simulink model "Control_UAV_Phat"  (R2016a)
settings: Solver=VariableStepAuto  StartTime=0.0  StopTime=30  RelTol=1e-3
PreLoadFcn:
  | parameters
InitFcn:
  | parameters
values from neighbouring files (symbols this model uses):
  attitudeInit = [0;0;0]    [parameters.m]
  b = 5.9347e-06    [parameters.m]
  d = 1.2181e-07    [parameters.m]
  g = 9.81    [parameters.m]
  I = diag([Ix,Iy,Iz])    [parameters.m]
  k1_pitch = kxip*wp_n*Iy/(Kth*L)    [parameters.m]
  k1_roll = kxir*wr_n*Ix/(Kth*L)    [parameters.m]
  k1_yaw = kxiy*wy_n*Iz/(2*Kd)    [parameters.m]
  k2_pitch = (wp_n^2)*Iy/(2*k1_pitch*Kth*L)    [parameters.m]
  k2_roll = (wr_n^2)*Ix/(2*k1_roll*Kth*L)    [parameters.m]
  k2_yaw = (wy_n^2)*Iz/(4*k1_yaw*Kd)    [parameters.m]
  kd_x = 4*g/(kxi_positionx*wposition_nx)    (= 29.0666666667)    [parameters.m]
  kd_y = 4*g/(kxi_positiony*wposition_ny)    (= 78.48)    [parameters.m]
  ki_h = 0.04    [parameters.m]
  kp_h = 2*wh_n*kxih*m/(4*Kth)    [parameters.m]
  kp_x = 2*g/wposition_nx^2    (= 8.72)    [parameters.m]
  kp_y = 2*g/wposition_ny^2    (= 19.62)    [parameters.m]
  Ks = 735    [parameters.m]
  L = 0.17    [parameters.m]
  m = 0.616    [parameters.m]
  omegaInit = [0;0;0]    [parameters.m]
  posInit = [0;0;0]    [parameters.m]
  tau = 1/200    (= 0.005)    [parameters.m]
  u0 = 0.49    [parameters.m]
  velInit = [0;0;0]    [parameters.m]
settings Model: Creator=Hiii  LastModifiedBy=Hii
settings GRTTargetCC: GeneratePreprocessorConditionals=Use local settings

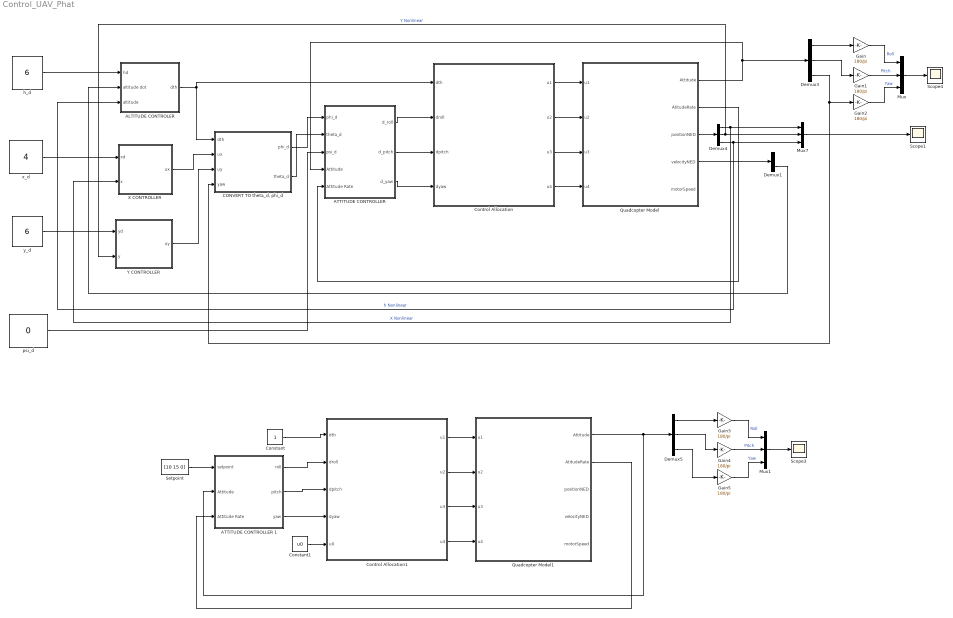
== system Control_UAV_Phat ==
  "ALTITUDE CONTROLER " : Subsystem
  "ATTITUDE CONTROLLER " : Subsystem
  ATTITUDE CONTROLLER 1 : Subsystem
  "CONVERT TO theta_d, phi_d " : MATLAB Function  TreatAsAtomicUnit=on
  Constant : Constant
  Constant1 : Constant  Value=u0
  Control Allocation : Subsystem
  Control Allocation1 : Subsystem
  Demux{1,3..5} (4 alike) : Demux  Outputs=3
  Gain{,1..5} (6 alike) : Gain  Gain=180/pi
  Mux : Mux  Inputs=3
  Mux1 : Mux  Inputs=3
  Mux7 : Mux  Inputs=3
  Quadcopter Model : Subsystem
  Quadcopter Model1 : Subsystem
  Scope1 : Scope
  Scope3 : Scope
  Scope4 : Scope
  "Setpoint " : Constant  Value=[10 15 0]
  "X CONTROLLER " : Subsystem
  "Y CONTROLLER " : Subsystem
  "h_d " : Constant  Value=6
  psi_d : Constant  Value=0
  "x_d " : Constant  Value=4
  "y_d " : Constant  Value=6
  wires:
  Demux3/3 -> Gain2/1, "CONVERT TO theta_d, phi_d "/4(yaw)
  Demux4/3 -> "ALTITUDE CONTROLER "/3("altitude "), Mux7/3  "h Nonlinear"
  Demux4/2 -> "Y CONTROLLER "/2(y), Mux7/2  "Y Nonlinear"
  Demux4/1 -> Mux7/1, "X CONTROLLER "/2(x)  "X Nonlinear"
  Quadcopter Model/3("positionNED ") -> Demux4/1
  Quadcopter Model/1(Attitude) -> "ATTITUDE CONTROLLER "/4("Attitude "), Demux3/1
  Quadcopter Model/4(velocityNED) -> Demux1/1
  "ALTITUDE CONTROLER "/1(dth) -> Control Allocation/1(dth), "CONVERT TO theta_d, phi_d "/1(dth)
  "X CONTROLLER "/1("ux ") -> "CONVERT TO theta_d, phi_d "/2(ux)
  "Y CONTROLLER "/1("uy ") -> "CONVERT TO theta_d, phi_d "/3(uy)
  "y_d "/1 -> "Y CONTROLLER "/1(yd)
  "x_d "/1 -> "X CONTROLLER "/1(xd)
  "h_d "/1 -> "ALTITUDE CONTROLER "/1(hd)
  Demux1/3 -> "ALTITUDE CONTROLER "/2("altitude dot ")
  Control Allocation/1("u1 ") -> Quadcopter Model/1("u1 ")
  Control Allocation/2("u2 ") -> Quadcopter Model/2("u2 ")
  Control Allocation/3("u3 ") -> Quadcopter Model/3("u3 ")
  Control Allocation/4("u4 ") -> Quadcopter Model/4("u4 ")
  "ATTITUDE CONTROLLER "/1("d_roll ") -> Control Allocation/2(droll)
  "ATTITUDE CONTROLLER "/2("d_pitch ") -> Control Allocation/3(dpitch)
  "ATTITUDE CONTROLLER "/3("d_yaw ") -> Control Allocation/4(dyaw)
  "CONVERT TO theta_d, phi_d "/1(phi_d) -> "ATTITUDE CONTROLLER "/1(phi_d)
  "CONVERT TO theta_d, phi_d "/2(theta_d) -> "ATTITUDE CONTROLLER "/2(theta_d)
  psi_d/1 -> "ATTITUDE CONTROLLER "/3("psi_d ")
  Quadcopter Model/2(AtitudeRate) -> "ATTITUDE CONTROLLER "/5("Attitude Rate ")
  Demux3/1 -> Gain/1
  Demux3/2 -> Gain1/1
  Mux/1 -> Scope4/1
  Gain/1 -> Mux/1  "Roll"
  Gain1/1 -> Mux/2  "Pitch"
  Gain2/1 -> Mux/3  "Yaw"
  Mux7/1 -> Scope1/1
  Demux5/3 -> Gain5/1
  Quadcopter Model1/1(Attitude) -> ATTITUDE CONTROLLER 1/2("Attitude "), Demux5/1
  Control Allocation1/1("u1 ") -> Quadcopter Model1/1("u1 ")
  Control Allocation1/2("u2 ") -> Quadcopter Model1/2("u2 ")
  Control Allocation1/3("u3 ") -> Quadcopter Model1/3("u3 ")
  Control Allocation1/4("u4 ") -> Quadcopter Model1/4("u4 ")
  ATTITUDE CONTROLLER 1/1("roll ") -> Control Allocation1/2(droll)
  ATTITUDE CONTROLLER 1/2("pitch ") -> Control Allocation1/3(dpitch)
  ATTITUDE CONTROLLER 1/3("yaw ") -> Control Allocation1/4(dyaw)
  Quadcopter Model1/2(AtitudeRate) -> ATTITUDE CONTROLLER 1/3("Attitude Rate ")
  Demux5/1 -> Gain3/1
  Demux5/2 -> Gain4/1
  Mux1/1 -> Scope3/1
  Gain3/1 -> Mux1/1  "Roll"
  Gain4/1 -> Mux1/2  "Pitch"
  Gain5/1 -> Mux1/3  "Yaw"
  Constant/1 -> Control Allocation1/1(dth)
  "Setpoint "/1 -> ATTITUDE CONTROLLER 1/1("setpoint ")
  Constant1/1 -> Control Allocation1/5("u0 ")

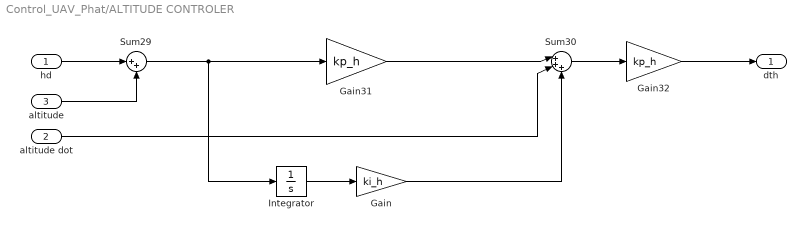
== system Control_UAV_Phat/ALTITUDE CONTROLER  ==
  hd : Inport  Description=hd
  "altitude dot " : Inport  Description=hd  Port=2
  "altitude " : Inport  Description=hd  Port=3
  Gain : Gain  Gain=ki_h
  Gain31 : Gain  Gain=kp_h
  Gain32 : Gain  Gain=kp_h
  Integrator : Integrator
  Sum29 : Sum  Inputs=|++
  Sum30 : Sum  Inputs=|+++
  dth : Outport
  wires:
  "altitude dot "/1 -> Sum30/2
  Sum30/1 -> Gain32/1
  Sum29/1 -> Integrator/1, Gain31/1
  hd/1 -> Sum29/1
  "altitude "/1 -> Sum29/2
  Gain32/1 -> dth/1
  Gain31/1 -> Sum30/1
  Integrator/1 -> Gain/1
  Gain/1 -> Sum30/3

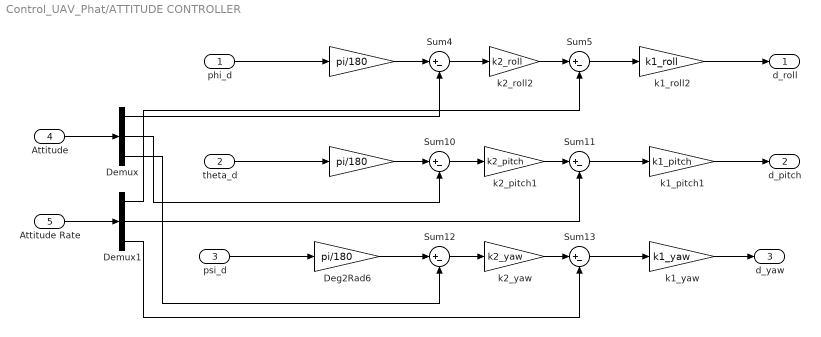
== system Control_UAV_Phat/ATTITUDE CONTROLLER  ==
  phi_d : Inport
  theta_d : Inport  Port=2
  "psi_d " : Inport  Port=3
  "Attitude " : Inport  Port=4
  "Attitude Rate " : Inport  Port=5
  " " : Gain  Gain=pi/180
  " " : Gain  Gain=pi/180
  Deg2Rad6 : Gain  Gain=pi/180
  Demux : Demux  Outputs=3
  Demux1 : Demux  Outputs=3
  Sum{4..5,10..13} (6 alike) : Sum  Inputs=|+-
  k1_pitch1 : Gain  Gain=k1_pitch
  k1_roll2 : Gain  Gain=k1_roll
  k1_yaw : Gain  Gain=k1_yaw
  k2_pitch1 : Gain  Gain=k2_pitch
  k2_roll2 : Gain  Gain=k2_roll
  k2_yaw : Gain  Gain=k2_yaw
  "d_roll " : Outport
  "d_pitch " : Outport  Port=2
  "d_yaw " : Outport  Port=3
  wires:
  k2_pitch1/1 -> Sum11/1
  Deg2Rad6/1 -> Sum12/1
  k2_yaw/1 -> Sum13/1
  " "/1 -> Sum4/1
  k2_roll2/1 -> Sum5/1
  Sum11/1 -> k1_pitch1/1
  Sum5/1 -> k1_roll2/1
  Sum10/1 -> k2_pitch1/1
  Sum4/1 -> k2_roll2/1
  " "/1 -> Sum10/1
  Sum12/1 -> k2_yaw/1
  Sum13/1 -> k1_yaw/1
  k1_roll2/1 -> "d_roll "/1
  k1_pitch1/1 -> "d_pitch "/1
  k1_yaw/1 -> "d_yaw "/1
  "Attitude "/1 -> Demux/1
  "Attitude Rate "/1 -> Demux1/1
  Demux/1 -> Sum4/2
  Demux/2 -> Sum10/2
  Demux/3 -> Sum12/2
  Demux1/1 -> Sum5/2
  Demux1/2 -> Sum11/2
  Demux1/3 -> Sum13/2
  phi_d/1 -> " "/1
  theta_d/1 -> " "/1
  "psi_d "/1 -> Deg2Rad6/1

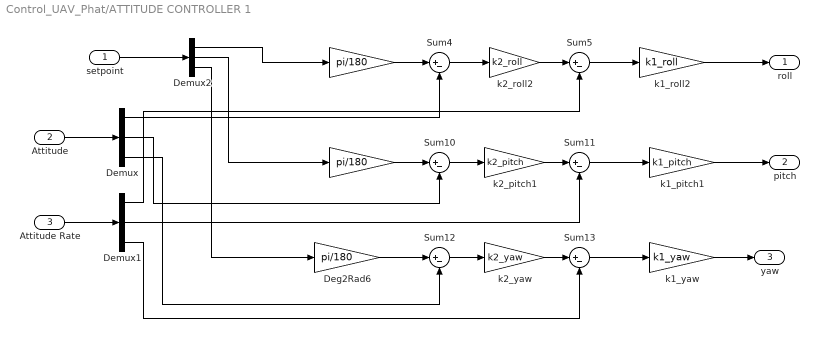
== system Control_UAV_Phat/ATTITUDE CONTROLLER 1 ==
  "setpoint " : Inport
  "Attitude " : Inport  Port=2
  "Attitude Rate " : Inport  Port=3
  " " : Gain  Gain=pi/180
  " " : Gain  Gain=pi/180
  Deg2Rad6 : Gain  Gain=pi/180
  Demux : Demux  Outputs=3
  Demux1 : Demux  Outputs=3
  Demux2 : Demux  Outputs=3
  Sum{4..5,10..13} (6 alike) : Sum  Inputs=|+-
  k1_pitch1 : Gain  Gain=k1_pitch
  k1_roll2 : Gain  Gain=k1_roll
  k1_yaw : Gain  Gain=k1_yaw
  k2_pitch1 : Gain  Gain=k2_pitch
  k2_roll2 : Gain  Gain=k2_roll
  k2_yaw : Gain  Gain=k2_yaw
  "roll " : Outport
  "pitch " : Outport  Port=2
  "yaw " : Outport  Port=3
  wires:
  k2_pitch1/1 -> Sum11/1
  Deg2Rad6/1 -> Sum12/1
  k2_yaw/1 -> Sum13/1
  " "/1 -> Sum4/1
  k2_roll2/1 -> Sum5/1
  Sum11/1 -> k1_pitch1/1
  Sum5/1 -> k1_roll2/1
  Sum10/1 -> k2_pitch1/1
  Sum4/1 -> k2_roll2/1
  " "/1 -> Sum10/1
  Sum12/1 -> k2_yaw/1
  Sum13/1 -> k1_yaw/1
  k1_roll2/1 -> "roll "/1
  k1_pitch1/1 -> "pitch "/1
  k1_yaw/1 -> "yaw "/1
  "Attitude "/1 -> Demux/1
  "Attitude Rate "/1 -> Demux1/1
  Demux/1 -> Sum4/2
  Demux/2 -> Sum10/2
  Demux/3 -> Sum12/2
  Demux1/1 -> Sum5/2
  Demux1/2 -> Sum11/2
  Demux1/3 -> Sum13/2
  "setpoint "/1 -> Demux2/1
  Demux2/1 -> " "/1
  Demux2/2 -> " "/1
  Demux2/3 -> Deg2Rad6/1

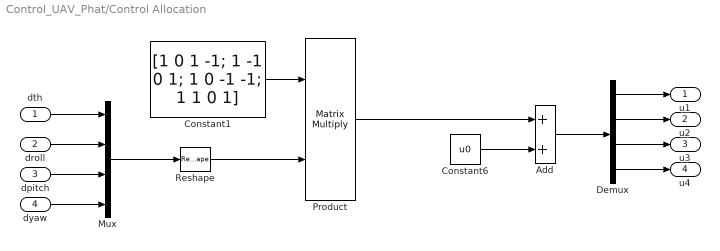
== system Control_UAV_Phat/Control Allocation ==
  dth : Inport
  droll : Inport  Port=2
  dpitch : Inport  Port=3
  dyaw : Inport  Port=4
  Add : Sum
  Constant1 : Constant  Value=[1 0 1 -1; 1 -1 0 1; 1 0 -1 -1; 1 1 0 1]
  Constant6 : Constant  Value=u0
  Demux : Demux
  Mux : Mux
  Product : Product  Multiplication=Matrix(*)
  Reshape : Reshape  OutputDimensionality=Column vector (2-D)
  "u1 " : Outport
  "u2 " : Outport  Port=2
  "u3 " : Outport  Port=3
  "u4 " : Outport  Port=4
  wires:
  Mux/1 -> Reshape/1
  dpitch/1 -> Mux/3
  dyaw/1 -> Mux/4
  Product/1 -> Add/1
  Reshape/1 -> Product/2
  Constant1/1 -> Product/1
  dth/1 -> Mux/1
  droll/1 -> Mux/2
  Constant6/1 -> Add/2
  Demux/1 -> "u1 "/1
  Demux/2 -> "u2 "/1
  Demux/3 -> "u3 "/1
  Demux/4 -> "u4 "/1
  Add/1 -> Demux/1

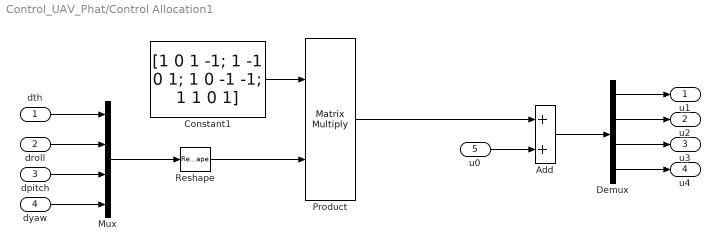
== system Control_UAV_Phat/Control Allocation1 ==
  dth : Inport
  droll : Inport  Port=2
  dpitch : Inport  Port=3
  dyaw : Inport  Port=4
  "u0 " : Inport  Port=5
  Add : Sum
  Constant1 : Constant  Value=[1 0 1 -1; 1 -1 0 1; 1 0 -1 -1; 1 1 0 1]
  Demux : Demux
  Mux : Mux
  Product : Product  Multiplication=Matrix(*)
  Reshape : Reshape  OutputDimensionality=Column vector (2-D)
  "u1 " : Outport
  "u2 " : Outport  Port=2
  "u3 " : Outport  Port=3
  "u4 " : Outport  Port=4
  wires:
  Mux/1 -> Reshape/1
  dpitch/1 -> Mux/3
  dyaw/1 -> Mux/4
  Product/1 -> Add/1
  Reshape/1 -> Product/2
  Constant1/1 -> Product/1
  dth/1 -> Mux/1
  droll/1 -> Mux/2
  Demux/1 -> "u1 "/1
  Demux/2 -> "u2 "/1
  Demux/3 -> "u3 "/1
  Demux/4 -> "u4 "/1
  Add/1 -> Demux/1
  "u0 "/1 -> Add/2

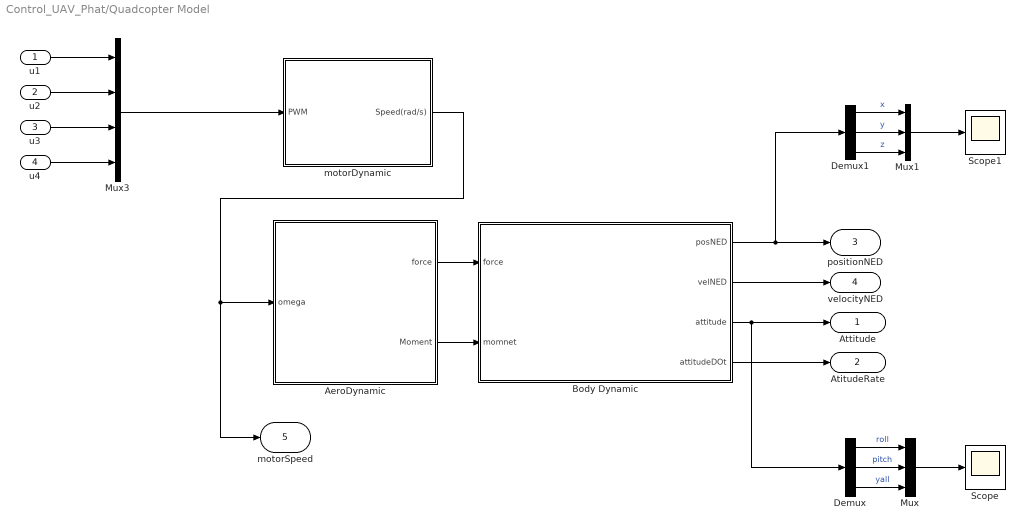
== system Control_UAV_Phat/Quadcopter Model ==
  "u1 " : Inport
  "u2 " : Inport  Port=2
  "u3 " : Inport  Port=3
  "u4 " : Inport  Port=4
  "AeroDynamic " : Subsystem
  "Body Dynamic " : Subsystem
  Demux : Demux  Outputs=3
  Demux1 : Demux  Outputs=3
  Mux : Mux  Inputs=3
  Mux1 : Mux  Inputs=3
  Mux3 : Mux
  Scope : Scope
  Scope1 : Scope
  "motorDynamic " : Subsystem
  Attitude : Outport
  AtitudeRate : Outport  Port=2
  "positionNED " : Outport  Port=3
  velocityNED : Outport  Port=4
  "motorSpeed " : Outport  Port=5
  wires:
  "AeroDynamic "/1(force) -> "Body Dynamic "/1("force ")
  "AeroDynamic "/2(Moment) -> "Body Dynamic "/2("momnet ")
  Demux/1 -> Mux/1  "roll"
  Demux/2 -> Mux/2  "pitch"
  Demux/3 -> Mux/3  "yall"
  Mux/1 -> Scope/1
  Demux1/1 -> Mux1/1  "x"
  Demux1/2 -> Mux1/2  "y"
  Demux1/3 -> Mux1/3  "z"
  Mux1/1 -> Scope1/1
  "Body Dynamic "/1(posNED) -> Demux1/1, "positionNED "/1
  "Body Dynamic "/3("attitude ") -> Demux/1, Attitude/1
  Mux3/1 -> "motorDynamic "/1("PWM ")
  "u1 "/1 -> Mux3/1
  "u2 "/1 -> Mux3/2
  "u3 "/1 -> Mux3/3
  "u4 "/1 -> Mux3/4
  "motorDynamic "/1("Speed(rad/s) ") -> "motorSpeed "/1, "AeroDynamic "/1("omega ")
  "Body Dynamic "/2(velNED) -> velocityNED/1
  "Body Dynamic "/4("attitudeDOt ") -> AtitudeRate/1

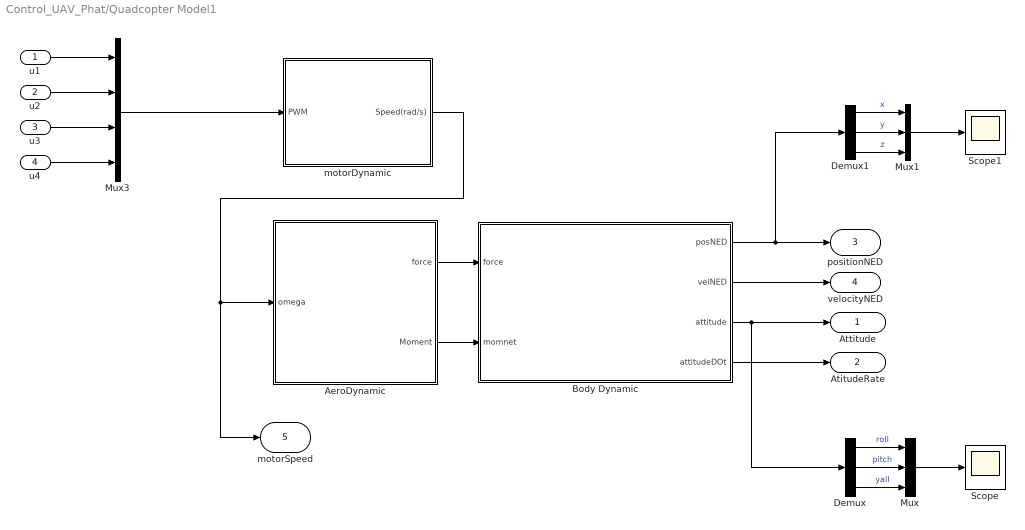
== system Control_UAV_Phat/Quadcopter Model1 ==
  "u1 " : Inport
  "u2 " : Inport  Port=2
  "u3 " : Inport  Port=3
  "u4 " : Inport  Port=4
  "AeroDynamic " : Subsystem
  "Body Dynamic " : Subsystem
  Demux : Demux  Outputs=3
  Demux1 : Demux  Outputs=3
  Mux : Mux  Inputs=3
  Mux1 : Mux  Inputs=3
  Mux3 : Mux
  Scope : Scope
  Scope1 : Scope
  "motorDynamic " : Subsystem
  Attitude : Outport
  AtitudeRate : Outport  Port=2
  "positionNED " : Outport  Port=3
  velocityNED : Outport  Port=4
  "motorSpeed " : Outport  Port=5
  wires:
  "AeroDynamic "/1(force) -> "Body Dynamic "/1("force ")
  "AeroDynamic "/2(Moment) -> "Body Dynamic "/2("momnet ")
  Demux/1 -> Mux/1  "roll"
  Demux/2 -> Mux/2  "pitch"
  Demux/3 -> Mux/3  "yall"
  Mux/1 -> Scope/1
  Demux1/1 -> Mux1/1  "x"
  Demux1/2 -> Mux1/2  "y"
  Demux1/3 -> Mux1/3  "z"
  Mux1/1 -> Scope1/1
  "Body Dynamic "/1(posNED) -> Demux1/1, "positionNED "/1
  "Body Dynamic "/3("attitude ") -> Demux/1, Attitude/1
  Mux3/1 -> "motorDynamic "/1("PWM ")
  "u1 "/1 -> Mux3/1
  "u2 "/1 -> Mux3/2
  "u3 "/1 -> Mux3/3
  "u4 "/1 -> Mux3/4
  "motorDynamic "/1("Speed(rad/s) ") -> "motorSpeed "/1, "AeroDynamic "/1("omega ")
  "Body Dynamic "/2(velNED) -> velocityNED/1
  "Body Dynamic "/4("attitudeDOt ") -> AtitudeRate/1

== system Control_UAV_Phat/X CONTROLLER  ==
  xd : Inport
  x : Inport  Port=2
  " " : Gain  Gain=kd_x
  Derivative4 : Derivative
  Gain1 : Gain  Gain=kp_x
  Sum1 : Sum  Inputs=|+-
  Sum2 : Sum  Inputs=|++
  "ux " : Outport
  wires:
  x/1 -> Sum1/2
  xd/1 -> Sum1/1
  Gain1/1 -> Sum2/1
  " "/1 -> Sum2/2
  Derivative4/1 -> " "/1
  Sum2/1 -> "ux "/1
  Sum1/1 -> Derivative4/1, Gain1/1

== system Control_UAV_Phat/Y CONTROLLER  ==
  yd : Inport
  y : Inport  Port=2
  " " : Gain  Gain=kd_y
  Derivative3 : Derivative
  Gain1 : Gain  Gain=kp_y
  Sum1 : Sum  Inputs=|+-
  Sum2 : Sum  Inputs=|++
  "uy " : Outport
  wires:
  Sum2/1 -> "uy "/1
  Sum1/1 -> Derivative3/1, Gain1/1
  Gain1/1 -> Sum2/1
  " "/1 -> Sum2/2
  yd/1 -> Sum1/1
  Derivative3/1 -> " "/1
  y/1 -> Sum1/2

== system Control_UAV_Phat/Quadcopter Model/AeroDynamic  ==
  "omega " : Inport
  "Area Dymanic " : MATLAB Function  TreatAsAtomicUnit=on
  Constant : Constant  Value=L
  Constant1 : Constant  Value=b
  Constant2 : Constant  Value=d
  force : Outport
  Moment : Outport  Port=2
  wires:
  "Area Dymanic "/1(force) -> force/1
  "Area Dymanic "/2(Moment) -> Moment/1
  Constant/1 -> "Area Dymanic "/2(L)
  Constant1/1 -> "Area Dymanic "/3(b)
  Constant2/1 -> "Area Dymanic "/4(d)
  "omega "/1 -> "Area Dymanic "/1(omega)

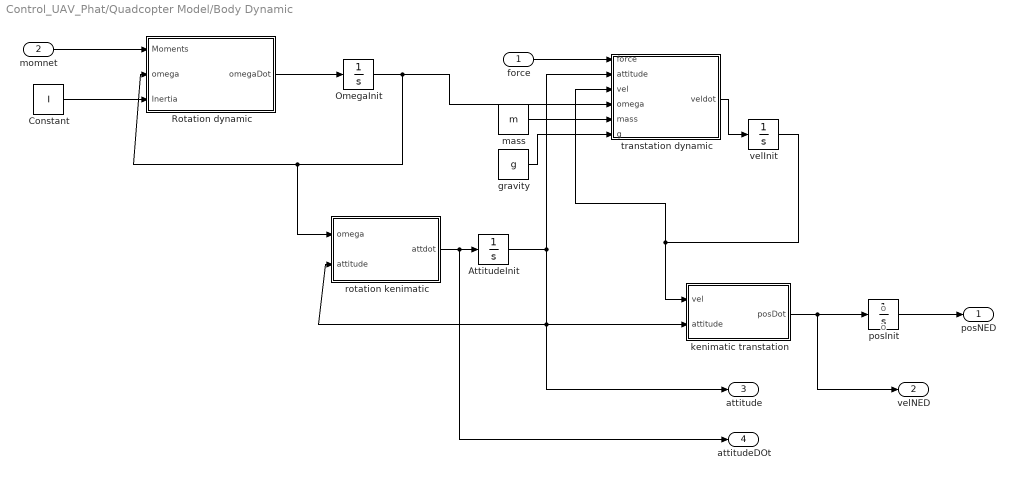
== system Control_UAV_Phat/Quadcopter Model/Body Dynamic  ==
  note: o
  note: o
  "force " : Inport
  "momnet " : Inport  Port=2
  "AttitudeInit " : Integrator  InitialCondition=attitudeInit
  Constant : Constant  Value=I
  "OmegaInit " : Integrator  InitialCondition=omegaInit
  "Rotation dynamic " : MATLAB Function  TreatAsAtomicUnit=on
  "gravity " : Constant  Value=g
  "kenimatic transtation " : MATLAB Function  TreatAsAtomicUnit=on
  mass : Constant  Value=m
  "posInit " : Integrator  InitialCondition=posInit
  "rotation kenimatic " : MATLAB Function  TreatAsAtomicUnit=on
  "transtation dynamic " : MATLAB Function  TreatAsAtomicUnit=on
  "velInit " : Integrator  InitialCondition=velInit
  posNED : Outport
  velNED : Outport  Port=2
  "attitude " : Outport  Port=3
  "attitudeDOt " : Outport  Port=4
  wires:
  "force "/1 -> "transtation dynamic "/1(force)
  mass/1 -> "transtation dynamic "/5(mass)
  "Rotation dynamic "/1(omegaDot) -> "OmegaInit "/1
  "OmegaInit "/1 -> "Rotation dynamic "/2(omega), "rotation kenimatic "/1(omega), "transtation dynamic "/4(omega)
  "momnet "/1 -> "Rotation dynamic "/1(Moments)
  Constant/1 -> "Rotation dynamic "/3(Inertia)
  "AttitudeInit "/1 -> "attitude "/1, "kenimatic transtation "/2(attitude), "rotation kenimatic "/2(attitude), "transtation dynamic "/2(attitude)
  "posInit "/1 -> posNED/1
  "rotation kenimatic "/1(attdot) -> "attitudeDOt "/1, "AttitudeInit "/1
  "kenimatic transtation "/1(posDot) -> velNED/1, "posInit "/1
  "gravity "/1 -> "transtation dynamic "/6(g)
  "velInit "/1 -> "kenimatic transtation "/1(vel), "transtation dynamic "/3(vel)
  "transtation dynamic "/1(veldot) -> "velInit "/1

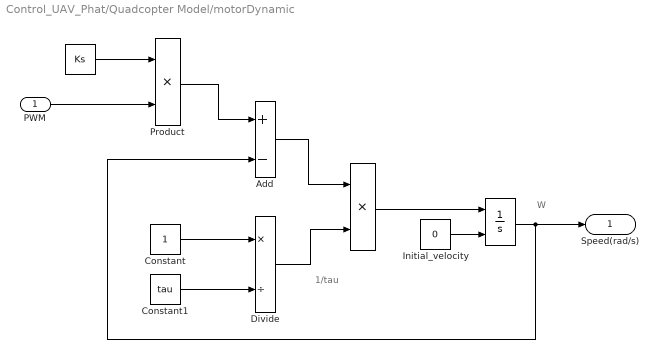
== system Control_UAV_Phat/Quadcopter Model/motorDynamic  ==
  note: 1/tau
  note: W
  "PWM " : Inport
  " " : Constant  Value=Ks
  " " : Product
  " " : Integrator  InitialConditionSource=external
  Add : Sum  Inputs=+-
  Constant : Constant
  Constant1 : Constant  Value=tau
  Divide : Product  Inputs=*/
  "Initial_velocity " : Constant  Value=0
  Product : Product
  "Speed(rad/s) " : Outport
  wires:
  " "/1 -> Product/1
  Product/1 -> Add/1
  "PWM "/1 -> Product/2
  Constant1/1 -> Divide/2
  Constant/1 -> Divide/1
  Add/1 -> " "/1
  Divide/1 -> " "/2
  " "/1 -> " "/1
  "Initial_velocity "/1 -> " "/2
  " "/1 -> Add/2, "Speed(rad/s) "/1

== system Control_UAV_Phat/Quadcopter Model1/AeroDynamic  ==
  "omega " : Inport
  "Area Dymanic " : MATLAB Function  TreatAsAtomicUnit=on
  Constant : Constant  Value=L
  Constant1 : Constant  Value=b
  Constant2 : Constant  Value=d
  force : Outport
  Moment : Outport  Port=2
  wires:
  "Area Dymanic "/1(force) -> force/1
  "Area Dymanic "/2(Moment) -> Moment/1
  Constant/1 -> "Area Dymanic "/2(L)
  Constant1/1 -> "Area Dymanic "/3(b)
  Constant2/1 -> "Area Dymanic "/4(d)
  "omega "/1 -> "Area Dymanic "/1(omega)

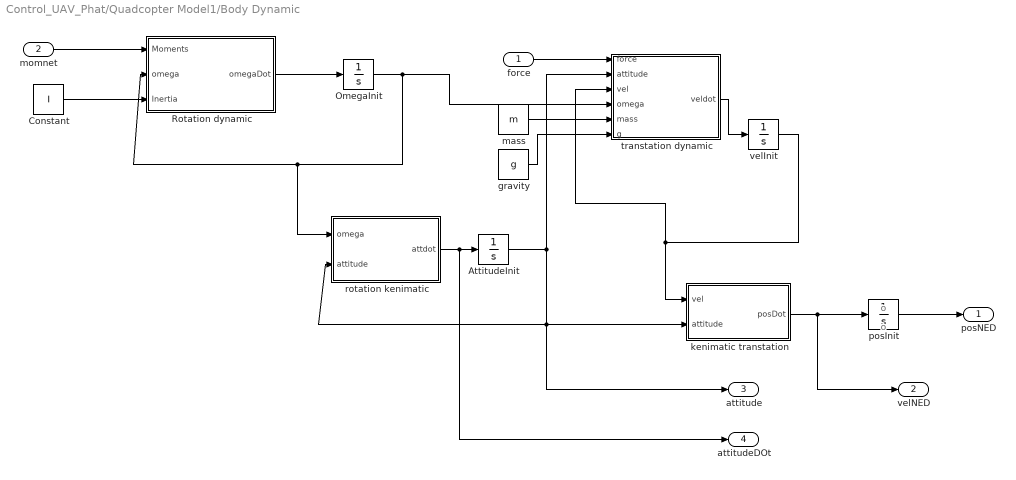
== system Control_UAV_Phat/Quadcopter Model1/Body Dynamic  ==
  note: o
  note: o
  "force " : Inport
  "momnet " : Inport  Port=2
  "AttitudeInit " : Integrator  InitialCondition=attitudeInit
  Constant : Constant  Value=I
  "OmegaInit " : Integrator  InitialCondition=omegaInit
  "Rotation dynamic " : MATLAB Function  TreatAsAtomicUnit=on
  "gravity " : Constant  Value=g
  "kenimatic transtation " : MATLAB Function  TreatAsAtomicUnit=on
  mass : Constant  Value=m
  "posInit " : Integrator  InitialCondition=posInit
  "rotation kenimatic " : MATLAB Function  TreatAsAtomicUnit=on
  "transtation dynamic " : MATLAB Function  TreatAsAtomicUnit=on
  "velInit " : Integrator  InitialCondition=velInit
  posNED : Outport
  velNED : Outport  Port=2
  "attitude " : Outport  Port=3
  "attitudeDOt " : Outport  Port=4
  wires:
  "force "/1 -> "transtation dynamic "/1(force)
  mass/1 -> "transtation dynamic "/5(mass)
  "Rotation dynamic "/1(omegaDot) -> "OmegaInit "/1
  "OmegaInit "/1 -> "Rotation dynamic "/2(omega), "rotation kenimatic "/1(omega), "transtation dynamic "/4(omega)
  "momnet "/1 -> "Rotation dynamic "/1(Moments)
  Constant/1 -> "Rotation dynamic "/3(Inertia)
  "AttitudeInit "/1 -> "attitude "/1, "kenimatic transtation "/2(attitude), "rotation kenimatic "/2(attitude), "transtation dynamic "/2(attitude)
  "posInit "/1 -> posNED/1
  "rotation kenimatic "/1(attdot) -> "attitudeDOt "/1, "AttitudeInit "/1
  "kenimatic transtation "/1(posDot) -> velNED/1, "posInit "/1
  "gravity "/1 -> "transtation dynamic "/6(g)
  "velInit "/1 -> "kenimatic transtation "/1(vel), "transtation dynamic "/3(vel)
  "transtation dynamic "/1(veldot) -> "velInit "/1

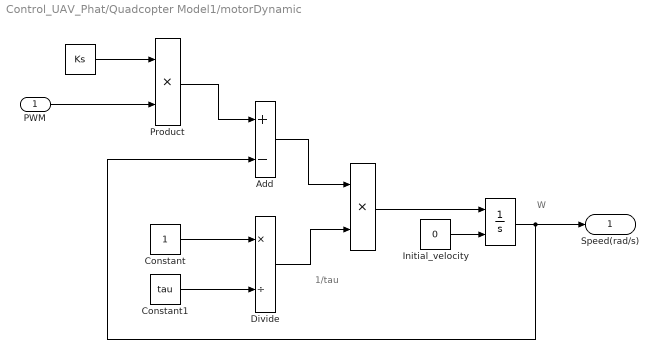
== system Control_UAV_Phat/Quadcopter Model1/motorDynamic  ==
  note: 1/tau
  note: W
  "PWM " : Inport
  " " : Constant  Value=Ks
  " " : Product
  " " : Integrator  InitialConditionSource=external
  Add : Sum  Inputs=+-
  Constant : Constant
  Constant1 : Constant  Value=tau
  Divide : Product  Inputs=*/
  "Initial_velocity " : Constant  Value=0
  Product : Product
  "Speed(rad/s) " : Outport
  wires:
  " "/1 -> Product/1
  Product/1 -> Add/1
  "PWM "/1 -> Product/2
  Constant1/1 -> Divide/2
  Constant/1 -> Divide/1
  Add/1 -> " "/1
  Divide/1 -> " "/2
  " "/1 -> " "/1
  "Initial_velocity "/1 -> " "/2
  " "/1 -> Add/2, "Speed(rad/s) "/1

== matlab function Control_UAV_Phat/Quadcopter Model1/AeroDynamic /Area Dymanic  ==
  data: omega input; force output; L input; b input; d input; Moment output
function [force,Moment] = fcn(omega,L,b,d)
%#codegen
omega1=omega(1);
omega2=omega(2);
omega3=omega(3);
omega4=omega(4);
F= b*(omega1^(2)+omega2^(2)+ omega3^(2)+ omega4^(2));
moment= [L*b*(omega4^(2)-omega2^(2));
        L*b*(omega1^(2)- omega3^(2));
        d*(-omega1^(2)+omega2^(2)-omega3^(2)+omega4^(2))];
force= [0;0;-F];        
Moment=moment;

== matlab function Control_UAV_Phat/Quadcopter Model1/Body Dynamic /Rotation dynamic  ==
  data: Moments input; omegaDot output; omega input; Inertia input
function omegaDot = fcn(Moments, omega, Inertia)
%#codegen 

omegaDot = Inertia^(-1)*(Moments-cross(omega,Inertia*omega));

== matlab function Control_UAV_Phat/Quadcopter Model1/Body Dynamic /kenimatic transtation  ==
  data: vel input; posDot output; attitude input
function posDot = fcn(vel,attitude)
phi = attitude(1);
theta = attitude(2);
psi= attitude(3);
R = [cos(theta)*cos(psi), cos(psi)*sin(phi)*sin(theta) - cos(phi)*sin(psi), sin(phi)*sin(psi) + cos(phi)*cos(psi)*sin(theta)
     cos(theta)*sin(psi), cos(phi)*cos(psi) + sin(phi)*sin(theta)*sin(psi), cos(phi)*sin(theta)*sin(psi) - cos(psi)*sin(phi)
             -sin(theta),                              cos(theta)*sin(phi),                            cos(phi)*cos(theta)];

%velocity output x_dot, y_dot, z_dot
posDot = R*vel;

== matlab function Control_UAV_Phat/Quadcopter Model1/Body Dynamic /rotation kenimatic  ==
  data: omega input; attdot output; attitude input
function attdot = fcn(omega,attitude)
phi = attitude(1);
theta = attitude(2);
psi= attitude(3);
W =[1 sin(phi)*tan(theta) cos(phi)*tan(theta);
   0 cos(phi) -sin(phi); 
   0 sin(phi)/cos(theta) cos(phi)/cos(theta)];
attdot = W*omega;

== matlab function Control_UAV_Phat/Quadcopter Model/AeroDynamic /Area Dymanic  ==
  data: omega input; force output; L input; b input; d input; Moment output
function [force,Moment] = fcn(omega,L,b,d)
%#codegen
omega1=omega(1);
omega2=omega(2);
omega3=omega(3);
omega4=omega(4);
F= b*(omega1^(2)+omega2^(2)+ omega3^(2)+ omega4^(2));
moment= [L*b*(omega4^(2)-omega2^(2));
        L*b*(omega1^(2)- omega3^(2));
        d*(-omega1^(2)+omega2^(2)-omega3^(2)+omega4^(2))];
force= [0;0;-F];        
Moment=moment;

== matlab function Control_UAV_Phat/Quadcopter Model/Body Dynamic /Rotation dynamic  ==
  data: Moments input; omegaDot output; omega input; Inertia input
function omegaDot = fcn(Moments, omega, Inertia)
%#codegen 

omegaDot = Inertia^(-1)*(Moments-cross(omega,Inertia*omega));

== matlab function Control_UAV_Phat/Quadcopter Model/Body Dynamic /kenimatic transtation  ==
  data: vel input; posDot output; attitude input
function posDot = fcn(vel,attitude)
phi = attitude(1);
theta = attitude(2);
psi= attitude(3);
R = [cos(theta)*cos(psi), cos(psi)*sin(phi)*sin(theta) - cos(phi)*sin(psi), sin(phi)*sin(psi) + cos(phi)*cos(psi)*sin(theta)
     cos(theta)*sin(psi), cos(phi)*cos(psi) + sin(phi)*sin(theta)*sin(psi), cos(phi)*sin(theta)*sin(psi) - cos(psi)*sin(phi)
             -sin(theta),                              cos(theta)*sin(phi),                            cos(phi)*cos(theta)];

%velocity output x_dot, y_dot, z_dot
posDot = R*vel;

== matlab function Control_UAV_Phat/Quadcopter Model/Body Dynamic /rotation kenimatic  ==
  data: omega input; attdot output; attitude input
function attdot = fcn(omega,attitude)
phi = attitude(1);
theta = attitude(2);
psi= attitude(3);
W =[1 sin(phi)*tan(theta) cos(phi)*tan(theta);
   0 cos(phi) -sin(phi); 
   0 sin(phi)/cos(theta) cos(phi)/cos(theta)];
attdot = W*omega;

== matlab function Control_UAV_Phat/Quadcopter Model/Body Dynamic /transtation dynamic  ==
  data: force input; veldot output; attitude input; vel input; omega input; mass input; g input
function veldot = fcn(force,attitude,vel,omega,mass,g)
phi = attitude(1);
theta = attitude(2);
G= [-g*sin(theta);g*sin(phi)*cos(theta);g*cos(phi)*cos(theta)];

veldot = 1/mass*force+G- cross(omega,vel);

== matlab function Control_UAV_Phat/Quadcopter Model1/Body Dynamic /transtation dynamic  ==
  data: force input; veldot output; attitude input; vel input; omega input; mass input; g input
function veldot = fcn(force,attitude,vel,omega,mass,g)
phi = attitude(1);
theta = attitude(2);
G= [-g*sin(theta);g*sin(phi)*cos(theta);g*cos(phi)*cos(theta)];

veldot = 1/mass*force+G- cross(omega,vel);

== matlab function Control_UAV_Phat/CONVERT TO theta_d, phi_d  ==
  data: dth input; ux input; phi_d output; uy input; yaw input; theta_d output
function [phi_d, theta_d] = fcn(dth, ux, uy, yaw)
g=9.81;
uz=dth+g;
ux=-ux;
uy = -uy;
phi_d = atan2(sin(yaw)*cos(yaw)*ux-cos(yaw)^2*uy, uz);
sin_theta_d = cos(yaw)^2*ux+sin(yaw)*cos(yaw)*uy/ uz;
sin_theta_d = max(min(sin_theta_d, 1), -1);
theta_d = asin(sin_theta_d);
